simulink model "VariableMotorModel"  (R2015b)
settings: Solver=VariableStepAuto  StartTime=0.0  StopTime=10.0  RelTol=1e-3
undefined symbols (not defined in the file): Initial, Motor, Uav
libraries: simulink_extras x1
settings Model: Creator=jban039  LastModifiedBy=jban039

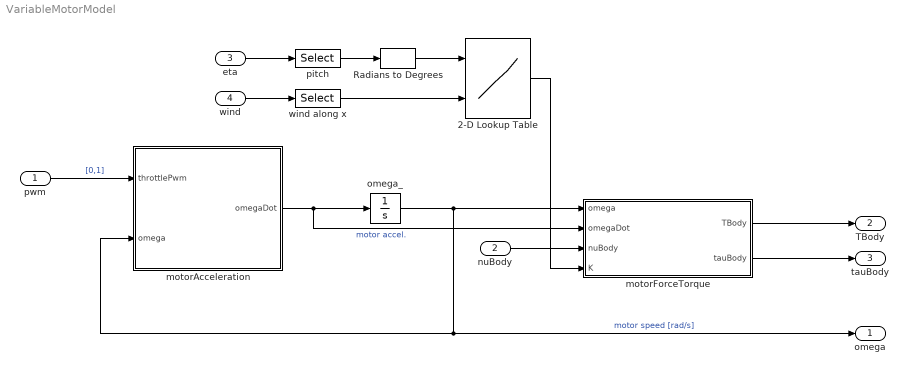
== system VariableMotorModel ==
  pwm : Inport  PortDimensions=Uav.N_ROTORS
  nuBody : Inport  Port=2
  eta : Inport  Port=3
  wind : Inport  Port=4
  2-D Lookup Table : Lookup_n-D  BreakpointsForDimension1=[0,2.890909,6.009259676377,9.296238414,12.27875]  BreakpointsForDimension2=[0,10,20]  Table=reshape([9.55641004221352e-06,1.00990801427108e-05,1.28091919414946e-05,1.45562427543497e-05,1.63017404112369e-05,1.00884339028815e-05,1.06718323589317e-05,1.12577089455794e-05,1.21229824131359e-05,1.24606394544993e-05,9.47230336229989e-06,9.71233115660863e-06,9.65341998978562e-06,9.60249125674676e-06,8.92828582195144e-06],5,3)  InternalRulePriority=Speed  RndMeth=Simplest  InputSameDT=on
  Radians to Degrees : simulink_extras/Transformations/Radians to Degrees
  motorAcceleration : MATLAB Function  TreatAsAtomicUnit=on
  motorForceTorque : MATLAB Function  TreatAsAtomicUnit=on
  omega_ : Integrator  InitialCondition=Initial.OMEGA
  pitch : Selector  InputPortWidth=3  IndexOptions=Index vector (dialog)  Indices=[2]  OutputSizes=1
  wind along x : Selector  InputPortWidth=3  IndexOptions=Index vector (dialog)  Indices=[1]  OutputSizes=1
  omega : Outport
  TBody : Outport  Port=2
  tauBody : Outport  Port=3
  wires:
  motorAcceleration/1(omegaDot) -> motorForceTorque/2(omegaDot), omega_/1  "motor accel."
  motorForceTorque/2(tauBody) -> tauBody/1
  motorForceTorque/1(TBody) -> TBody/1
  omega_/1 -> motorAcceleration/2(omega), omega/1, motorForceTorque/1(omega)  "motor speed [rad/s]"
  pwm/1 -> motorAcceleration/1(throttlePwm)  "[0,1]"
  nuBody/1 -> motorForceTorque/3(nuBody)
  wind along x/1 -> 2-D Lookup Table/2
  pitch/1 -> Radians to Degrees/1
  wind/1 -> wind along x/1
  eta/1 -> pitch/1
  2-D Lookup Table/1 -> motorForceTorque/4(K)
  Radians to Degrees/1 -> 2-D Lookup Table/1

== matlab function VariableMotorModel/motorForceTorque ==
  data: omega input; TBody output size=3; omegaDot input; nuBody input size=3; Motor parameter; Uav parameter; tauBody output size=3; K input
function [TBody, tauBody] = motorForceTorque(...
    omega, omegaDot, nuBody, Motor, Uav, K)
%#codegen

% Make assertions to avoid code generation errors
assert(Uav.N_ROTORS < 16);

%% Thrust and differential torque

% Concatenated motor force/torque vectors in respective motor frame
% eg. TMotor = [TMotor1, TMotor2, ..., TMotorN]
% where: - N is the number of rotors
%        - TMotorx (x ∈ [1,2,...,N]) is the thrust generated by motor x in
%          its own frame of reference
TMotorIndividual = [ zeros(2, Uav.N_ROTORS);
                     K * (omega'.^2) ];
tauMotorIndividual = [ zeros(2, Uav.N_ROTORS);
                      -Uav.ROTOR_DIRECTION .* ...
                 ( Motor.B*(omega'.^2) + Motor.I_R(3,3)*omegaDot' ) ];

% Initialise matrices to store motor force/torque vectors in body frame
TBodyIndividual   = zeros(3, Uav.N_ROTORS);
tauBodyIndividual = zeros(3, Uav.N_ROTORS);

% Calculate forces and moments from each motor in the body frame
for i = 1:Uav.N_ROTORS
    l = Uav.L(i);
    beta = Uav.BETA(i);
    
    % Matrix to compute torque applied by rotor thrust
 	L = [ 0,            0,            l*sin(beta);
          0,            0,           -l*cos(beta);
         -l*sin(beta),  l*cos(beta),  0 ];

	% Motor force/torque vectors in body frame
	TBodyIndividual(:,i) = Uav.R_MOTOR_TO_BODY(:,:,i) * ...
        TMotorIndividual(:,i);
	tauBodyIndividual(:,i) = Uav.R_MOTOR_TO_BODY(:,:,i) * ...
        tauMotorIndividual(:,i) + L * TBodyIndividual(:,i);
end

%% Gyroscopic moments

% Concatenated gyroscopic moments for each rotor
M_GBodyIndividual = zeros(3, Uav.N_ROTORS);

% Concatenated motor speeds in their respective frames
omegaMotor = [ zeros(2, Uav.N_ROTORS);
               Uav.ROTOR_DIRECTION .* omega' ];

% Angular momentum in motor frame
H_MMotorSeparate = Motor.I_R * omegaMotor;

% Gyroscopic moment vectors in body frame
for i = 1:Uav.N_ROTORS
	M_GBodyIndividual(:,i) = cross( nuBody, ...
        Uav.R_MOTOR_TO_BODY(:,:,i) * H_MMotorSeparate(:,i) );
end

M_GBody = sum(M_GBodyIndividual, 2);

%% Total torque and moment

% Total force/torque in body frame
TBody = sum(TBodyIndividual, 2);
tauBody = sum(tauBodyIndividual, 2) - M_GBody;

end

== matlab function VariableMotorModel/motorAcceleration ==
  data: throttlePwm input; omegaDot output double size=4; omega input; Motor parameter; Uav parameter
function omegaDot = motorAcceleration(throttlePwm, omega, Motor, Uav)
%#codegen

voltage = throttlePwm * Uav.NOMINAL_BATTERY_VOLTAGE;

% Motor current ignoring inductance
current = (voltage - Motor.K_E*omega) / Motor.R;

netTorque = (Motor.K_T * current) - (Motor.B * omega.^2);

% Motor angular acceleration
omegaDot = netTorque / Motor.I_R(3,3);
